simulink model "mpc_switching_explicit"  (R2023a)
settings: Solver=ode45  StartTime=0.0  StopTime=100  FixedStep=1e-5  RelTol=1e-3
values from neighbouring files (symbols this model uses):
  b1 = 0.3    [ScheduleControllersAtMultipleOperatingPoints1.m]
  b2 = 0.8    [ScheduleControllersAtMultipleOperatingPoints1.m]
  k1 = 1    [ScheduleControllersAtMultipleOperatingPoints1.m]
  k2 = 0.1    [ScheduleControllersAtMultipleOperatingPoints1.m]
  M1 = 1    [ScheduleControllersAtMultipleOperatingPoints1.m]
  M2 = 5    [ScheduleControllersAtMultipleOperatingPoints1.m]
  y1initial = 0    [ScheduleControllersAtMultipleOperatingPoints1.m]
  y2initial = 10    [ScheduleControllersAtMultipleOperatingPoints1.m]
  yeq1 = 10    [ScheduleControllersAtMultipleOperatingPoints1.m]
  yeq2 = -10    [ScheduleControllersAtMultipleOperatingPoints1.m]
libraries: simulink x4, mpclib x1
settings Model: ExtModeTrigMode=oneshot  Creator=The MathWorks, Inc.  LastModifiedBy=The MathWorks, Inc.
settings SolverCC: AlgebraicLoopSolver=TrustRegion  InsertRTBMode=Auto  MaxZcPerStep=1
settings DataIOCC: SaveFormat=Array  ReturnWorkspaceOutputs=off  SignalLoggingName=sigsOut
settings OptimizationCC: BooleanDataType=off  ExpressionDepthLimit=2147483647  InitFltsAndDblsToZero=on  EfficientMapNaN2IntZero=off  LifeSpan=inf
settings DebuggingCC: SaveWithParameterizedLinksMsg=none  UnderspecifiedInitializationDetection=Classic  MergeDetectMultiDrivingBlocksExec=none  CheckExecutionContextPreStartOutputMsg=on  SignalResolutionControl=TryResolveAllWithWarning  MultiTaskDSMMsg=warning  MultiTaskCondExecSysMsg=none  IntegerOverflowMsg=none  FcnCallInpInsideContextMsg=warning  UnconnectedInputMsg=warning  UnconnectedOutputMsg=warning  UnconnectedLineMsg=warning  StateNameClashWarn=warning  SubsystemReferenceDiagnosticForUnitTest=warning  SFUnexpectedBacktrackingDiag=warning  SFNoUnconditionalDefaultTransitionDiag=warning  SFExecutionAtInitializationDiag=none  IntegerSaturationMsg=none  ArithmeticOperatorsInVariantConditions=warning
settings HardwareCC: ProdBitPerPointer=32  ProdBitPerSizeT=32  ProdBitPerPtrDiffT=32  ProdLargestAtomicFloat=None  ProdIntDivRoundTo=Undefined  ProdEndianess=Unspecified  ProdWordSize=32  ProdHWDeviceType=32-bit Generic  TargetBitPerLong=64  TargetBitPerPointer=64  TargetBitPerSizeT=64  TargetBitPerPtrDiffT=64  TargetLongLongMode=on  TargetIntDivRoundTo=Zero  TargetEndianess=LittleEndian  TargetWordSize=64  TargetHWDeviceType=MATLAB Host  ProdEqTarget=off
settings ModelReferenceCC: EnableRefExpFcnMdlSchedulingChecks=on  PropagateSignalLabelsOutOfModel=off
settings SFSimCC: SimUseLocalCustomCode=off  CustomCodeUndefinedFunction=UseInterfaceOnly
settings RTWCC: RTWUseLocalCustomCode=off
settings CodeAppCC: StateflowObjectComments=on
settings GRTTargetCC: TargetFcnLib=ansi_tfl_tmw.mat  TargetLangStandard=C89/C90 (ANSI)  CombineOutputUpdateFcns=off  GRTInterface=on
settings ConfigComp: CovMetricSettings=dw  CovSaveCumulativeToWorkspaceVar=on  CovSaveSingleToWorkspaceVar=on  CovExternalEMLEnable=off  CovSFcnEnable=off

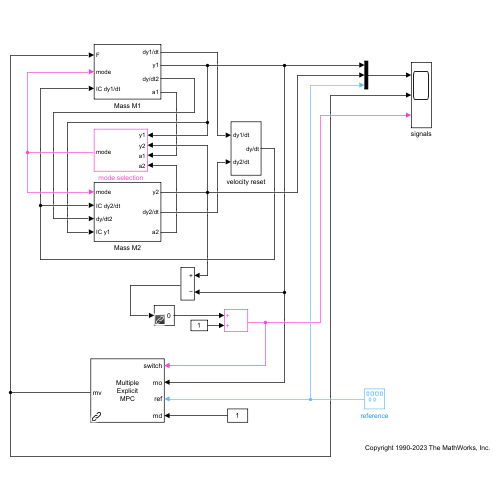
[thumbnail: Simulink's stored preview of the top-level diagram]
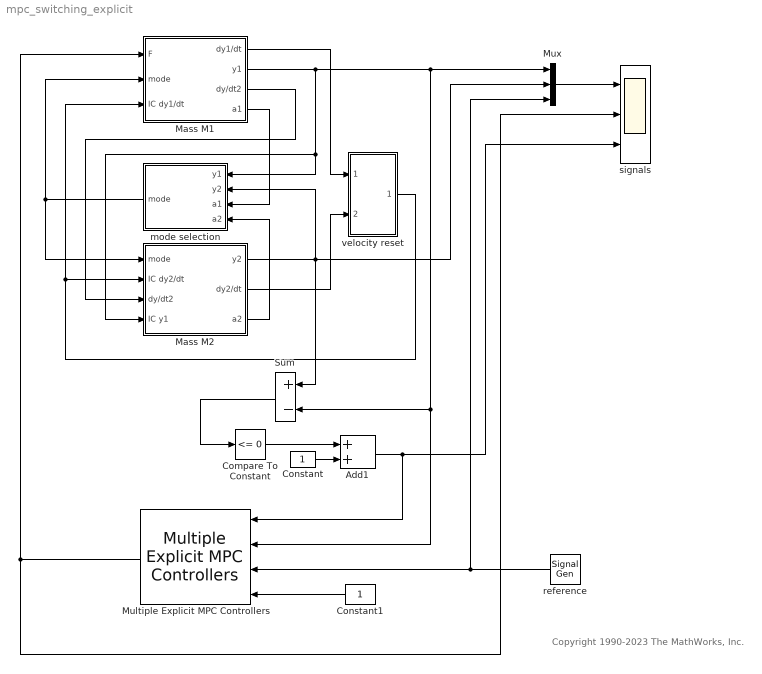
== system mpc_switching_explicit ==
  note: Copyright 1990-2023 The MathWorks, Inc.
  Add1 : Sum
  Compare To Constant : simulink/Logic and Bit Operations/Compare To Constant  relop=<=  const=0  OutDataTypeStr=uint8  ZeroCross=off
  Constant : Constant
  Constant1 : Constant
  Mass M1 : Subsystem
  Mass M2 : Subsystem
  Multiple Explicit MPC Controllers : mpclib/Multiple Explicit MPC Controllers  empcobjs={'expMPC1','expMPC2'}  x0s={'[]','[]'}  Nempc=1  theEMPC=1  nmv=1  nmo=1  nmd=1  nts=1  md_inport_multiple=on  mv_inport_multiple=off  return_status_multiple=off  return_region_multiple=off  return_state_multiple=off  state_inport_multiple=off  BlockDataType_multiple=double  SampleTimeInherited_multiple=off
  Mux : Mux  Inputs=3
  Sum : Sum  Inputs=+-
  mode selection : Subsystem
  reference : SignalGenerator  WaveForm=square  Amplitude=5  Frequency=.015
  signals : Scope  NumInputPorts=3
  velocity reset : Subsystem
  wires:
  Mass M1/1(dy1/dt) -> velocity reset/1(dy1/dt)
  Mass M2/1(y2) -> mode selection/2(y2), Sum/1, Mux/2
  Mass M1/2(y1) -> Mux/1, Multiple Explicit MPC Controllers/2, Sum/2, mode selection/1(y1), Mass M2/4(IC y1)
  mode selection/1(mode) -> Mass M1/2(mode), Mass M2/1(mode)
  Mass M2/2(dy2/dt) -> velocity reset/2(dy2/dt)
  velocity reset/1(dy/dt) -> Mass M2/2(IC dy2/dt), Mass M1/3(IC dy1/dt)
  Mux/1 -> signals/1
  Constant/1 -> Add1/2
  Constant1/1 -> Multiple Explicit MPC Controllers/4
  Multiple Explicit MPC Controllers/1 -> Mass M1/1(F), signals/2
  Mass M1/3(dy/dt2) -> Mass M2/3(dy/dt2)
  Add1/1 -> Multiple Explicit MPC Controllers/1, signals/3
  reference/1 -> Multiple Explicit MPC Controllers/3, Mux/3
  Mass M1/4(a1) -> mode selection/3(a1)
  Mass M2/3(a2) -> mode selection/4(a2)
  Compare To Constant/1 -> Add1/1
  Sum/1 -> Compare To Constant/1

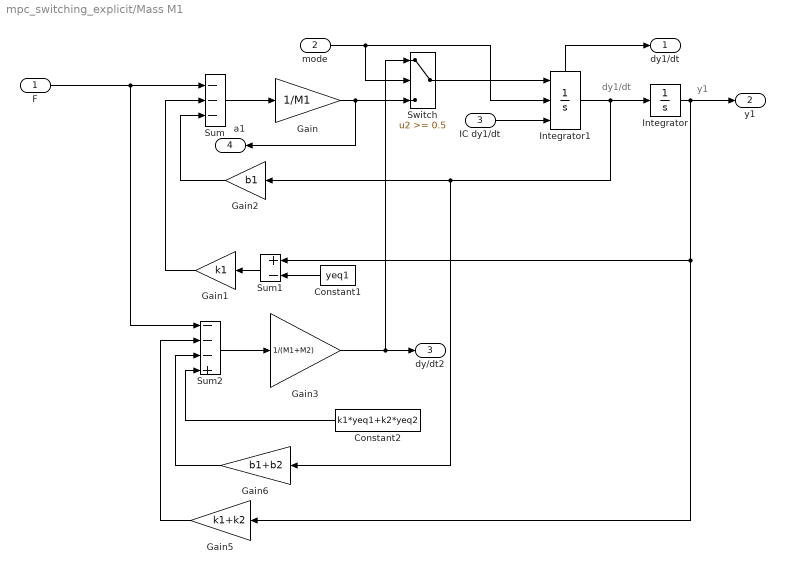
== system mpc_switching_explicit/Mass M1 ==
  note: y1
  note: dy1/dt
  F : Inport
  mode : Inport  Port=2
  IC dy1/dt : Inport  Port=3
  Constant1 : Constant  Value=yeq1
  Constant2 : Constant  Value=k1*yeq1+k2*yeq2
  Gain : Gain  Gain=1/M1
  Gain1 : Gain  Gain=k1
  Gain2 : Gain  Gain=b1
  Gain3 : Gain  Gain=1/(M1+M2)
  Gain5 : Gain  Gain=k1+k2
  Gain6 : Gain  Gain=b1+b2
  Integrator : Integrator  InitialCondition=y1initial
  Integrator1 : Integrator  ExternalReset=rising  InitialConditionSource=external  ShowStatePort=on
  Sum : Sum  Inputs=---
  Sum1 : Sum  Inputs=+-
  Sum2 : Sum  Inputs=---+
  Switch : Switch  Threshold=0.5  SaturateOnIntegerOverflow=off  InputSameDT=off
  dy1/dt : Outport
  y1 : Outport  Port=2
  dy/dt2 : Outport  Port=3
  a1 : Outport  Port=4
  wires:
  Integrator/1 -> Sum1/1, Gain5/1, y1/1
  Integrator1/1 -> Integrator/1, Gain2/1, Gain6/1
  Constant1/1 -> Sum1/2
  Sum1/1 -> Gain1/1
  Gain1/1 -> Sum/2
  Gain2/1 -> Sum/3
  F/1 -> Sum/1, Sum2/1
  mode/1 -> Integrator1/2, Switch/2
  Switch/1 -> Integrator1/1
  Sum/1 -> Gain/1
  Gain5/1 -> Sum2/2
  Gain6/1 -> Sum2/3
  Sum2/1 -> Gain3/1
  Constant2/1 -> Sum2/4
  Gain3/1 -> Switch/1, dy/dt2/1
  Gain/1 -> Switch/3, a1/1
  IC dy1/dt/1 -> Integrator1/3
  Integrator1/State -> dy1/dt/1

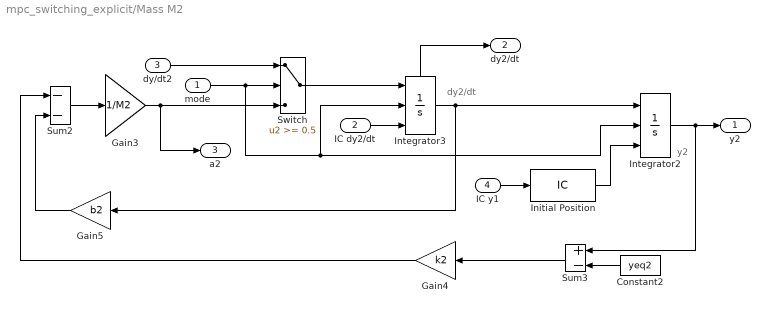
== system mpc_switching_explicit/Mass M2 ==
  note: dy2/dt
  note: y2
  mode : Inport
  IC dy2/dt : Inport  Port=2
  dy/dt2 : Inport  Port=3
  IC y1 : Inport  Port=4
  Constant2 : Constant  Value=yeq2
  Gain3 : Gain  Gain=1/M2
  Gain4 : Gain  Gain=k2
  Gain5 : Gain  Gain=b2
  Initial Position : InitialCondition  Value=y2initial
  Integrator2 : Integrator  ExternalReset=rising  InitialConditionSource=external  InitialCondition=y2initial
  Integrator3 : Integrator  ExternalReset=rising  InitialConditionSource=external  ShowStatePort=on
  Sum2 : Sum  Inputs=--
  Sum3 : Sum  Inputs=+-
  Switch : Switch  Threshold=0.5  SaturateOnIntegerOverflow=off  InputSameDT=off
  y2 : Outport
  dy2/dt : Outport  Port=2
  a2 : Outport  Port=3
  wires:
  Gain4/1 -> Sum2/1
  Gain5/1 -> Sum2/2
  Sum3/1 -> Gain4/1
  Constant2/1 -> Sum3/2
  Sum2/1 -> Gain3/1
  Integrator3/1 -> Gain5/1, Integrator2/1
  Integrator3/State -> dy2/dt/1
  Integrator2/1 -> Sum3/1, y2/1
  Switch/1 -> Integrator3/1
  mode/1 -> Integrator3/2, Integrator2/2, Switch/2
  Gain3/1 -> Switch/3, a2/1
  dy/dt2/1 -> Switch/1
  Initial Position/1 -> Integrator2/3
  IC y1/1 -> Initial Position/1
  IC dy2/dt/1 -> Integrator3/3

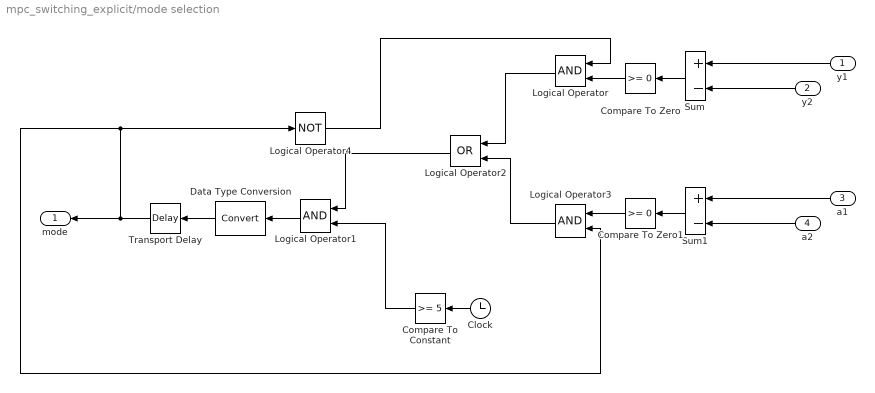
== system mpc_switching_explicit/mode selection ==
  y1 : Inport
  y2 : Inport  Port=2
  a1 : Inport  Port=3
  a2 : Inport  Port=4
  Clock : Clock
  Compare To Constant : simulink/Logic and Bit Operations/Compare To Constant  relop=>=  const=5  OutDataTypeStr=uint8  ZeroCross=off
  Compare To Zero : simulink/Logic and Bit Operations/Compare To Zero  relop=>=  OutDataTypeStr=boolean  ZeroCross=off
  Compare To Zero1 : simulink/Logic and Bit Operations/Compare To Zero  relop=>=  OutDataTypeStr=boolean  ZeroCross=off
  Data Type Conversion : DataTypeConversion  SaturateOnIntegerOverflow=off  RndMeth=Floor
  Logical Operator : Logic  AllPortsSameDT=off  OutDataTypeStr=boolean
  Logical Operator1 : Logic  AllPortsSameDT=off  OutDataTypeStr=boolean
  Logical Operator2 : Logic  Operator=OR  AllPortsSameDT=off  OutDataTypeStr=boolean
  Logical Operator3 : Logic  AllPortsSameDT=off  OutDataTypeStr=boolean
  Logical Operator4 : Logic  Operator=NOT  AllPortsSameDT=off  OutDataTypeStr=boolean
  Sum : Sum  Inputs=+-
  Sum1 : Sum  Inputs=+-
  Transport Delay : TransportDelay  DelayTime=1e-6
  mode : Outport
  wires:
  y1/1 -> Sum/1
  y2/1 -> Sum/2
  Sum/1 -> Compare To Zero/1
  a1/1 -> Sum1/1
  a2/1 -> Sum1/2
  Sum1/1 -> Compare To Zero1/1
  Transport Delay/1 -> mode/1, Logical Operator3/2, Logical Operator4/1
  Logical Operator4/1 -> Logical Operator/1
  Compare To Zero/1 -> Logical Operator/2
  Logical Operator/1 -> Logical Operator2/1
  Logical Operator3/1 -> Logical Operator2/2
  Compare To Zero1/1 -> Logical Operator3/1
  Clock/1 -> Compare To Constant/1
  Logical Operator2/1 -> Logical Operator1/1
  Compare To Constant/1 -> Logical Operator1/2
  Logical Operator1/1 -> Data Type Conversion/1
  Data Type Conversion/1 -> Transport Delay/1

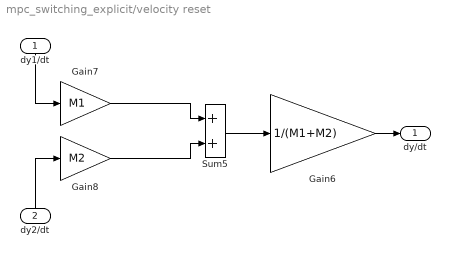
== system mpc_switching_explicit/velocity reset ==
  dy1/dt : Inport
  dy2/dt : Inport  Port=2
  Gain6 : Gain  Gain=1/(M1+M2)
  Gain7 : Gain  Gain=M1
  Gain8 : Gain  Gain=M2
  Sum5 : Sum
  dy/dt : Outport
  wires:
  Sum5/1 -> Gain6/1
  Gain7/1 -> Sum5/1
  Gain8/1 -> Sum5/2
  dy1/dt/1 -> Gain7/1
  dy2/dt/1 -> Gain8/1
  Gain6/1 -> dy/dt/1
